simulink model "lab7_1"  (R2018b)
settings: Solver=VariableStepAuto  StartTime=0.0  StopTime=10.0  RelTol=1e-3
libraries: hdlsllib x86
(part 1 of 2)
settings Model: Creator=Patrick  LastModifiedBy=Patrick

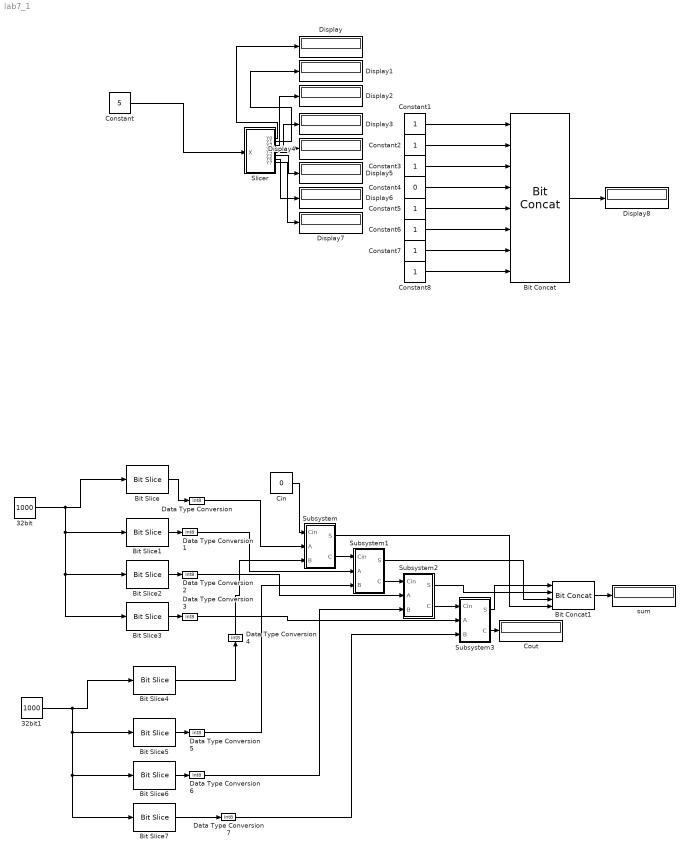
== system lab7_1 ==
  32bit : Constant  Value=1000  OutDataTypeStr=int32  SampleTime=1
  32bit1 : Constant  Value=1000  OutDataTypeStr=int32  SampleTime=1
  Bit Concat : hdlsllib/Logic and Bit Operations/Bit Concat  numInputs=8
      settings: SourceProductName=HDL Coder  SourceProductBaseCode=HD
  Bit Concat1 : hdlsllib/Logic and Bit Operations/Bit Concat  numInputs=4
      settings: SourceProductName=HDL Coder  SourceProductBaseCode=HD
  Bit Slice : hdlsllib/Logic and Bit Operations/Bit Slice  lidx=7  ridx=0
  Bit Slice1 : hdlsllib/Logic and Bit Operations/Bit Slice  lidx=15  ridx=8
  Bit Slice2 : hdlsllib/Logic and Bit Operations/Bit Slice  lidx=23  ridx=16
  Bit Slice3 : hdlsllib/Logic and Bit Operations/Bit Slice  lidx=31  ridx=24
  Bit Slice4 : hdlsllib/Logic and Bit Operations/Bit Slice  lidx=7  ridx=0
  Bit Slice5 : hdlsllib/Logic and Bit Operations/Bit Slice  lidx=15  ridx=8
  Bit Slice6 : hdlsllib/Logic and Bit Operations/Bit Slice  lidx=23  ridx=16
  Bit Slice7 : hdlsllib/Logic and Bit Operations/Bit Slice  lidx=31  ridx=24
  Cin : Constant  Value=0  OutDataTypeStr=boolean  SampleTime=1
  Constant : Constant  Value=5  OutDataTypeStr=int8
  Constant{1..3,5..8} (7 alike) : Constant  OutDataTypeStr=boolean
  Constant4 : Constant  Value=0  OutDataTypeStr=boolean
  Cout : Display
  Data Type Conversion{,1..7} (8 alike) : DataTypeConversion  OutDataTypeStr=int8
  Display{,1..8} (9 alike) : Display
  Slicer : Subsystem
  Subsystem : Subsystem
  Subsystem1 : Subsystem
  Subsystem2 : Subsystem
  Subsystem3 : Subsystem
  sum : Display
  wires:
  Constant/1 -> Slicer/1(X)
  Slicer/8(Y7) -> Display7/1
  Slicer/7(Y6) -> Display6/1
  Slicer/6(Y5) -> Display5/1
  Slicer/5(Y4) -> Display4/1
  Slicer/4(Y3) -> Display3/1
  Slicer/3(Y2) -> Display2/1
  Slicer/2(Y1) -> Display1/1
  Slicer/1(Y0) -> Display/1
  Constant1/1 -> Bit Concat/1
  Constant2/1 -> Bit Concat/2
  Constant3/1 -> Bit Concat/3
  Constant4/1 -> Bit Concat/4
  Constant5/1 -> Bit Concat/5
  Constant6/1 -> Bit Concat/6
  Constant7/1 -> Bit Concat/7
  Constant8/1 -> Bit Concat/8
  Bit Concat/1 -> Display8/1
  32bit/1 -> Bit Slice3/1, Bit Slice2/1, Bit Slice1/1, Bit Slice/1
  Bit Slice/1 -> Data Type Conversion/1
  Bit Slice2/1 -> Data Type Conversion2/1
  Bit Slice3/1 -> Data Type Conversion3/1
  Subsystem2/2(C) -> Subsystem3/1(Cin)
  Subsystem1/2(C) -> Subsystem2/1(Cin)
  Subsystem/2(C) -> Subsystem1/1(Cin)
  Bit Slice4/1 -> Data Type Conversion4/1
  32bit1/1 -> Bit Slice7/1, Bit Slice6/1, Bit Slice5/1, Bit Slice4/1
  Bit Slice7/1 -> Data Type Conversion7/1
  Subsystem3/1(S) -> Bit Concat1/1
  Subsystem2/1(S) -> Bit Concat1/2
  Subsystem1/1(S) -> Bit Concat1/3
  Subsystem/1(S) -> Bit Concat1/4
  Subsystem3/2(C) -> Cout/1
  Bit Concat1/1 -> sum/1
  Cin/1 -> Subsystem/1(Cin)
  Data Type Conversion/1 -> Subsystem/2(A)
  Data Type Conversion7/1 -> Subsystem3/3(B)
  Bit Slice6/1 -> Data Type Conversion6/1
  Data Type Conversion6/1 -> Subsystem2/3(B)
  Bit Slice5/1 -> Data Type Conversion5/1
  Data Type Conversion5/1 -> Subsystem1/3(B)
  Data Type Conversion4/1 -> Subsystem/3(B)
  Data Type Conversion3/1 -> Subsystem3/2(A)
  Data Type Conversion2/1 -> Subsystem2/2(A)
  Bit Slice1/1 -> Data Type Conversion1/1
  Data Type Conversion1/1 -> Subsystem1/2(A)

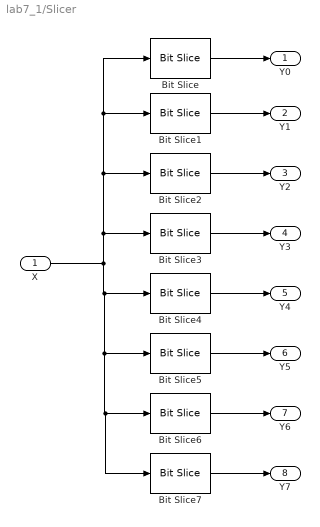
== system lab7_1/Slicer ==
  X : Inport  OutDataTypeStr=int8  SampleTime=1
  Bit Slice : hdlsllib/Logic and Bit Operations/Bit Slice  lidx=7  ridx=7
  Bit Slice1 : hdlsllib/Logic and Bit Operations/Bit Slice  lidx=6  ridx=6
  Bit Slice2 : hdlsllib/Logic and Bit Operations/Bit Slice  lidx=5  ridx=5
  Bit Slice3 : hdlsllib/Logic and Bit Operations/Bit Slice  lidx=4  ridx=4
  Bit Slice4 : hdlsllib/Logic and Bit Operations/Bit Slice  lidx=3  ridx=3
  Bit Slice5 : hdlsllib/Logic and Bit Operations/Bit Slice  lidx=2  ridx=2
  Bit Slice6 : hdlsllib/Logic and Bit Operations/Bit Slice  lidx=1  ridx=1
  Bit Slice7 : hdlsllib/Logic and Bit Operations/Bit Slice  lidx=0  ridx=0
  Y0 : Outport
  Y1 : Outport  Port=2
  Y2 : Outport  Port=3
  Y3 : Outport  Port=4
  Y4 : Outport  Port=5
  Y5 : Outport  Port=6
  Y6 : Outport  Port=7
  Y7 : Outport  Port=8
  wires:
  Bit Slice1/1 -> Y1/1
  Bit Slice7/1 -> Y7/1
  X/1 -> Bit Slice7/1, Bit Slice6/1, Bit Slice5/1, Bit Slice4/1, Bit Slice3/1, Bit Slice2/1, Bit Slice1/1, Bit Slice/1
  Bit Slice/1 -> Y0/1
  Bit Slice4/1 -> Y4/1
  Bit Slice2/1 -> Y2/1
  Bit Slice5/1 -> Y5/1
  Bit Slice3/1 -> Y3/1
  Bit Slice6/1 -> Y6/1

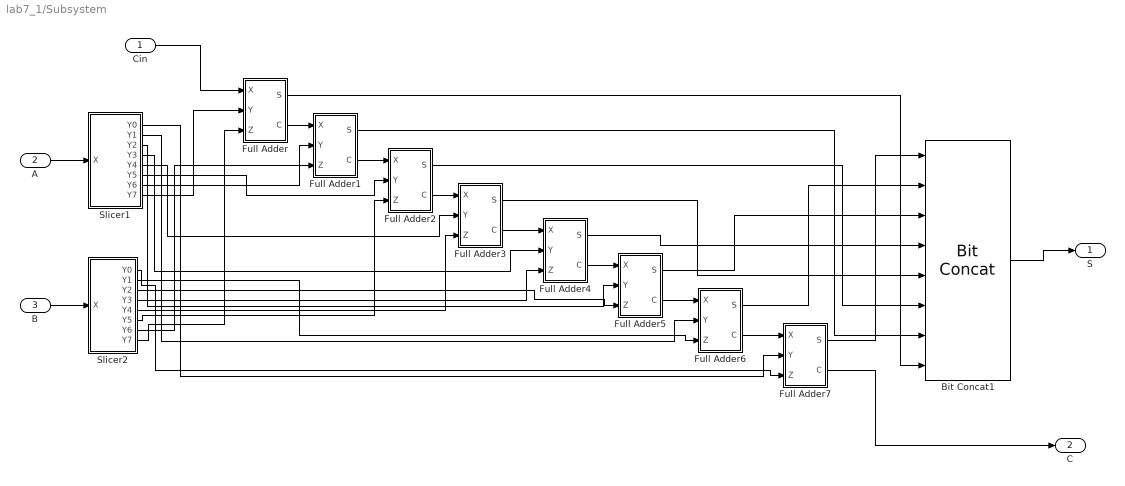
== system lab7_1/Subsystem ==
  Cin : Inport
  A : Inport  Port=2  OutDataTypeStr=int8
  B : Inport  Port=3  OutDataTypeStr=int8
  Bit Concat1 : hdlsllib/Logic and Bit Operations/Bit Concat  numInputs=8
      settings: SourceProductName=HDL Coder  SourceProductBaseCode=HD
  Full Adder : Subsystem
  Full Adder1 : Subsystem
  Full Adder2 : Subsystem
  Full Adder3 : Subsystem
  Full Adder4 : Subsystem
  Full Adder5 : Subsystem
  Full Adder6 : Subsystem
  Full Adder7 : Subsystem
  Slicer1 : Subsystem
  Slicer2 : Subsystem
  S : Outport
  C : Outport  Port=2
  wires:
  Full Adder/1(S) -> Bit Concat1/8
  A/1 -> Slicer1/1(X)
  Slicer1/8(Y7) -> Full Adder/2(Y)
  Cin/1 -> Full Adder/1(X)
  Full Adder4/2(C) -> Full Adder5/1(X)
  Slicer2/1(Y0) -> Full Adder7/3(Z)
  B/1 -> Slicer2/1(X)
  Slicer1/4(Y3) -> Full Adder4/2(Y)
  Slicer2/8(Y7) -> Full Adder/3(Z)
  Full Adder5/1(S) -> Bit Concat1/3
  Full Adder3/2(C) -> Full Adder4/1(X)
  Full Adder5/2(C) -> Full Adder6/1(X)
  Full Adder4/1(S) -> Bit Concat1/4
  Full Adder6/1(S) -> Bit Concat1/2
  Full Adder7/2(C) -> C/1
  Bit Concat1/1 -> S/1
  Slicer2/6(Y5) -> Full Adder2/3(Z)
  Slicer2/4(Y3) -> Full Adder4/3(Z)
  Full Adder7/1(S) -> Bit Concat1/1
  Full Adder/2(C) -> Full Adder1/1(X)
  Full Adder2/2(C) -> Full Adder3/1(X)
  Full Adder6/2(C) -> Full Adder7/1(X)
  Slicer1/5(Y4) -> Full Adder3/2(Y)
  Full Adder3/1(S) -> Bit Concat1/5
  Slicer2/7(Y6) -> Full Adder1/3(Z)
  Slicer2/2(Y1) -> Full Adder6/3(Z)
  Slicer1/1(Y0) -> Full Adder7/2(Y)
  Slicer2/5(Y4) -> Full Adder3/3(Z)
  Full Adder1/2(C) -> Full Adder2/1(X)
  Full Adder2/1(S) -> Bit Concat1/6
  Slicer1/6(Y5) -> Full Adder2/2(Y)
  Full Adder1/1(S) -> Bit Concat1/7
  Slicer1/3(Y2) -> Full Adder5/2(Y)
  Slicer1/7(Y6) -> Full Adder1/2(Y)
  Slicer2/3(Y2) -> Full Adder5/3(Z)
  Slicer1/2(Y1) -> Full Adder6/2(Y)

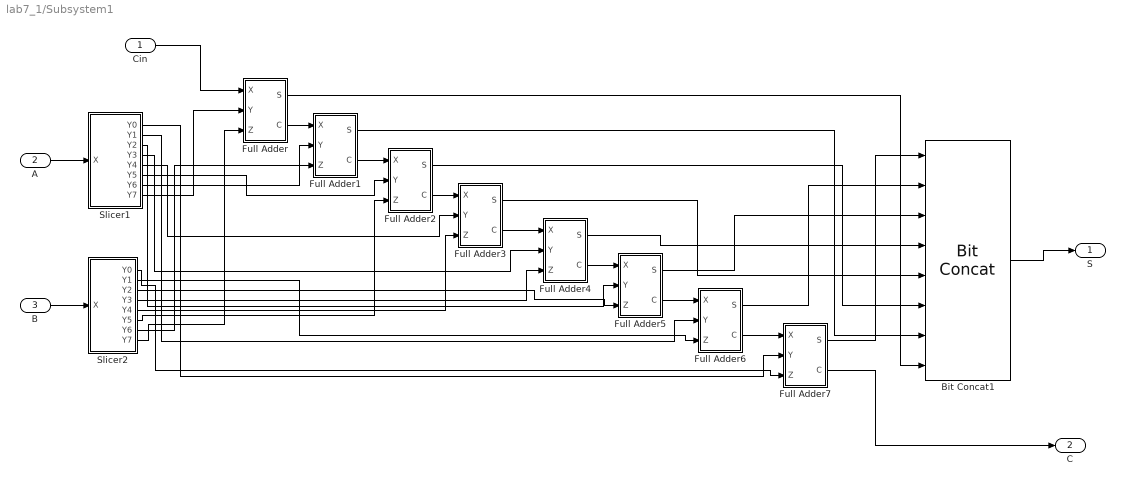
== system lab7_1/Subsystem1 ==
  Cin : Inport
  A : Inport  Port=2
  B : Inport  Port=3
  Bit Concat1 : hdlsllib/Logic and Bit Operations/Bit Concat  numInputs=8
      settings: SourceProductName=HDL Coder  SourceProductBaseCode=HD
  Full Adder : Subsystem
  Full Adder1 : Subsystem
  Full Adder2 : Subsystem
  Full Adder3 : Subsystem
  Full Adder4 : Subsystem
  Full Adder5 : Subsystem
  Full Adder6 : Subsystem
  Full Adder7 : Subsystem
  Slicer1 : Subsystem
  Slicer2 : Subsystem
  S : Outport
  C : Outport  Port=2
  wires:
  Full Adder/1(S) -> Bit Concat1/8
  A/1 -> Slicer1/1(X)
  Slicer1/8(Y7) -> Full Adder/2(Y)
  Cin/1 -> Full Adder/1(X)
  Full Adder4/2(C) -> Full Adder5/1(X)
  Slicer2/1(Y0) -> Full Adder7/3(Z)
  B/1 -> Slicer2/1(X)
  Slicer1/4(Y3) -> Full Adder4/2(Y)
  Slicer2/8(Y7) -> Full Adder/3(Z)
  Full Adder5/1(S) -> Bit Concat1/3
  Full Adder3/2(C) -> Full Adder4/1(X)
  Full Adder5/2(C) -> Full Adder6/1(X)
  Full Adder4/1(S) -> Bit Concat1/4
  Full Adder6/1(S) -> Bit Concat1/2
  Full Adder7/2(C) -> C/1
  Bit Concat1/1 -> S/1
  Slicer2/6(Y5) -> Full Adder2/3(Z)
  Slicer2/4(Y3) -> Full Adder4/3(Z)
  Full Adder7/1(S) -> Bit Concat1/1
  Full Adder/2(C) -> Full Adder1/1(X)
  Full Adder2/2(C) -> Full Adder3/1(X)
  Full Adder6/2(C) -> Full Adder7/1(X)
  Slicer1/5(Y4) -> Full Adder3/2(Y)
  Full Adder3/1(S) -> Bit Concat1/5
  Slicer2/7(Y6) -> Full Adder1/3(Z)
  Slicer2/2(Y1) -> Full Adder6/3(Z)
  Slicer1/1(Y0) -> Full Adder7/2(Y)
  Slicer2/5(Y4) -> Full Adder3/3(Z)
  Full Adder1/2(C) -> Full Adder2/1(X)
  Full Adder2/1(S) -> Bit Concat1/6
  Slicer1/6(Y5) -> Full Adder2/2(Y)
  Full Adder1/1(S) -> Bit Concat1/7
  Slicer1/3(Y2) -> Full Adder5/2(Y)
  Slicer1/7(Y6) -> Full Adder1/2(Y)
  Slicer2/3(Y2) -> Full Adder5/3(Z)
  Slicer1/2(Y1) -> Full Adder6/2(Y)

== system lab7_1/Subsystem2 ==
  Cin : Inport
  A : Inport  Port=2
  B : Inport  Port=3
  Bit Concat1 : hdlsllib/Logic and Bit Operations/Bit Concat  numInputs=8
      settings: SourceProductName=HDL Coder  SourceProductBaseCode=HD
  Full Adder : Subsystem
  Full Adder1 : Subsystem
  Full Adder2 : Subsystem
  Full Adder3 : Subsystem
  Full Adder4 : Subsystem
  Full Adder5 : Subsystem
  Full Adder6 : Subsystem
  Full Adder7 : Subsystem
  Slicer1 : Subsystem
  Slicer2 : Subsystem
  S : Outport
  C : Outport  Port=2
  wires:
  Full Adder/1(S) -> Bit Concat1/8
  A/1 -> Slicer1/1(X)
  Slicer1/8(Y7) -> Full Adder/2(Y)
  Cin/1 -> Full Adder/1(X)
  Full Adder4/2(C) -> Full Adder5/1(X)
  Slicer2/1(Y0) -> Full Adder7/3(Z)
  B/1 -> Slicer2/1(X)
  Slicer1/4(Y3) -> Full Adder4/2(Y)
  Slicer2/8(Y7) -> Full Adder/3(Z)
  Full Adder5/1(S) -> Bit Concat1/3
  Full Adder3/2(C) -> Full Adder4/1(X)
  Full Adder5/2(C) -> Full Adder6/1(X)
  Full Adder4/1(S) -> Bit Concat1/4
  Full Adder6/1(S) -> Bit Concat1/2
  Full Adder7/2(C) -> C/1
  Bit Concat1/1 -> S/1
  Slicer2/6(Y5) -> Full Adder2/3(Z)
  Slicer2/4(Y3) -> Full Adder4/3(Z)
  Full Adder7/1(S) -> Bit Concat1/1
  Full Adder/2(C) -> Full Adder1/1(X)
  Full Adder2/2(C) -> Full Adder3/1(X)
  Full Adder6/2(C) -> Full Adder7/1(X)
  Slicer1/5(Y4) -> Full Adder3/2(Y)
  Full Adder3/1(S) -> Bit Concat1/5
  Slicer2/7(Y6) -> Full Adder1/3(Z)
  Slicer2/2(Y1) -> Full Adder6/3(Z)
  Slicer1/1(Y0) -> Full Adder7/2(Y)
  Slicer2/5(Y4) -> Full Adder3/3(Z)
  Full Adder1/2(C) -> Full Adder2/1(X)
  Full Adder2/1(S) -> Bit Concat1/6
  Slicer1/6(Y5) -> Full Adder2/2(Y)
  Full Adder1/1(S) -> Bit Concat1/7
  Slicer1/3(Y2) -> Full Adder5/2(Y)
  Slicer1/7(Y6) -> Full Adder1/2(Y)
  Slicer2/3(Y2) -> Full Adder5/3(Z)
  Slicer1/2(Y1) -> Full Adder6/2(Y)

== system lab7_1/Subsystem3 ==
  Cin : Inport
  A : Inport  Port=2
  B : Inport  Port=3
  Bit Concat1 : hdlsllib/Logic and Bit Operations/Bit Concat  numInputs=8
      settings: SourceProductName=HDL Coder  SourceProductBaseCode=HD
  Full Adder : Subsystem
  Full Adder1 : Subsystem
  Full Adder2 : Subsystem
  Full Adder3 : Subsystem
  Full Adder4 : Subsystem
  Full Adder5 : Subsystem
  Full Adder6 : Subsystem
  Full Adder7 : Subsystem
  Slicer1 : Subsystem
  Slicer2 : Subsystem
  S : Outport
  C : Outport  Port=2
  wires:
  Full Adder/1(S) -> Bit Concat1/8
  A/1 -> Slicer1/1(X)
  Slicer1/8(Y7) -> Full Adder/2(Y)
  Cin/1 -> Full Adder/1(X)
  Full Adder4/2(C) -> Full Adder5/1(X)
  Slicer2/1(Y0) -> Full Adder7/3(Z)
  B/1 -> Slicer2/1(X)
  Slicer1/4(Y3) -> Full Adder4/2(Y)
  Slicer2/8(Y7) -> Full Adder/3(Z)
  Full Adder5/1(S) -> Bit Concat1/3
  Full Adder3/2(C) -> Full Adder4/1(X)
  Full Adder5/2(C) -> Full Adder6/1(X)
  Full Adder4/1(S) -> Bit Concat1/4
  Full Adder6/1(S) -> Bit Concat1/2
  Full Adder7/2(C) -> C/1
  Bit Concat1/1 -> S/1
  Slicer2/6(Y5) -> Full Adder2/3(Z)
  Slicer2/4(Y3) -> Full Adder4/3(Z)
  Full Adder7/1(S) -> Bit Concat1/1
  Full Adder/2(C) -> Full Adder1/1(X)
  Full Adder2/2(C) -> Full Adder3/1(X)
  Full Adder6/2(C) -> Full Adder7/1(X)
  Slicer1/5(Y4) -> Full Adder3/2(Y)
  Full Adder3/1(S) -> Bit Concat1/5
  Slicer2/7(Y6) -> Full Adder1/3(Z)
  Slicer2/2(Y1) -> Full Adder6/3(Z)
  Slicer1/1(Y0) -> Full Adder7/2(Y)
  Slicer2/5(Y4) -> Full Adder3/3(Z)
  Full Adder1/2(C) -> Full Adder2/1(X)
  Full Adder2/1(S) -> Bit Concat1/6
  Slicer1/6(Y5) -> Full Adder2/2(Y)
  Full Adder1/1(S) -> Bit Concat1/7
  Slicer1/3(Y2) -> Full Adder5/2(Y)
  Slicer1/7(Y6) -> Full Adder1/2(Y)
  Slicer2/3(Y2) -> Full Adder5/3(Z)
  Slicer1/2(Y1) -> Full Adder6/2(Y)

== system lab7_1/Subsystem/Full Adder ==
  X : Inport
  Y : Inport  Port=2
  Z : Inport  Port=3
  Half Adder : Subsystem
  Half Adder 1 : Subsystem
  Logical Operator : Logic  Operator=OR  IconShape=distinctive  AllPortsSameDT=off  OutDataTypeStr=boolean
  S : Outport
  C : Outport  Port=2
  wires:
  Half Adder/1(S) -> Half Adder 1/1(X)
  Y/1 -> Half Adder/2(Y)
  Half Adder 1/2(C) -> Logical Operator/1
  Z/1 -> Half Adder 1/2(Y)
  Half Adder/2(C) -> Logical Operator/2
  X/1 -> Half Adder/1(X)
  Half Adder 1/1(S) -> S/1
  Logical Operator/1 -> C/1

== system lab7_1/Subsystem/Full Adder1 ==
  X : Inport
  Y : Inport  Port=2
  Z : Inport  Port=3
  Half Adder : Subsystem
  Half Adder 1 : Subsystem
  Logical Operator : Logic  Operator=OR  IconShape=distinctive  AllPortsSameDT=off  OutDataTypeStr=boolean
  S : Outport
  C : Outport  Port=2
  wires:
  Half Adder/1(S) -> Half Adder 1/1(X)
  Y/1 -> Half Adder/2(Y)
  Half Adder 1/2(C) -> Logical Operator/1
  Z/1 -> Half Adder 1/2(Y)
  Half Adder/2(C) -> Logical Operator/2
  X/1 -> Half Adder/1(X)
  Half Adder 1/1(S) -> S/1
  Logical Operator/1 -> C/1

== system lab7_1/Subsystem/Full Adder2 ==
  X : Inport
  Y : Inport  Port=2
  Z : Inport  Port=3
  Half Adder : Subsystem
  Half Adder 1 : Subsystem
  Logical Operator : Logic  Operator=OR  IconShape=distinctive  AllPortsSameDT=off  OutDataTypeStr=boolean
  S : Outport
  C : Outport  Port=2
  wires:
  Half Adder/1(S) -> Half Adder 1/1(X)
  Y/1 -> Half Adder/2(Y)
  Half Adder 1/2(C) -> Logical Operator/1
  Z/1 -> Half Adder 1/2(Y)
  Half Adder/2(C) -> Logical Operator/2
  X/1 -> Half Adder/1(X)
  Half Adder 1/1(S) -> S/1
  Logical Operator/1 -> C/1

== system lab7_1/Subsystem/Full Adder3 ==
  X : Inport
  Y : Inport  Port=2
  Z : Inport  Port=3
  Half Adder : Subsystem
  Half Adder 1 : Subsystem
  Logical Operator : Logic  Operator=OR  IconShape=distinctive  AllPortsSameDT=off  OutDataTypeStr=boolean
  S : Outport
  C : Outport  Port=2
  wires:
  Half Adder/1(S) -> Half Adder 1/1(X)
  Y/1 -> Half Adder/2(Y)
  Half Adder 1/2(C) -> Logical Operator/1
  Z/1 -> Half Adder 1/2(Y)
  Half Adder/2(C) -> Logical Operator/2
  X/1 -> Half Adder/1(X)
  Half Adder 1/1(S) -> S/1
  Logical Operator/1 -> C/1

== system lab7_1/Subsystem/Full Adder4 ==
  X : Inport
  Y : Inport  Port=2
  Z : Inport  Port=3
  Half Adder : Subsystem
  Half Adder 1 : Subsystem
  Logical Operator : Logic  Operator=OR  IconShape=distinctive  AllPortsSameDT=off  OutDataTypeStr=boolean
  S : Outport
  C : Outport  Port=2
  wires:
  Half Adder/1(S) -> Half Adder 1/1(X)
  Y/1 -> Half Adder/2(Y)
  Half Adder 1/2(C) -> Logical Operator/1
  Z/1 -> Half Adder 1/2(Y)
  Half Adder/2(C) -> Logical Operator/2
  X/1 -> Half Adder/1(X)
  Half Adder 1/1(S) -> S/1
  Logical Operator/1 -> C/1

== system lab7_1/Subsystem/Full Adder5 ==
  X : Inport
  Y : Inport  Port=2
  Z : Inport  Port=3
  Half Adder : Subsystem
  Half Adder 1 : Subsystem
  Logical Operator : Logic  Operator=OR  IconShape=distinctive  AllPortsSameDT=off  OutDataTypeStr=boolean
  S : Outport
  C : Outport  Port=2
  wires:
  Half Adder/1(S) -> Half Adder 1/1(X)
  Y/1 -> Half Adder/2(Y)
  Half Adder 1/2(C) -> Logical Operator/1
  Z/1 -> Half Adder 1/2(Y)
  Half Adder/2(C) -> Logical Operator/2
  X/1 -> Half Adder/1(X)
  Half Adder 1/1(S) -> S/1
  Logical Operator/1 -> C/1

== system lab7_1/Subsystem/Full Adder6 ==
  X : Inport
  Y : Inport  Port=2
  Z : Inport  Port=3
  Half Adder : Subsystem
  Half Adder 1 : Subsystem
  Logical Operator : Logic  Operator=OR  IconShape=distinctive  AllPortsSameDT=off  OutDataTypeStr=boolean
  S : Outport
  C : Outport  Port=2
  wires:
  Half Adder/1(S) -> Half Adder 1/1(X)
  Y/1 -> Half Adder/2(Y)
  Half Adder 1/2(C) -> Logical Operator/1
  Z/1 -> Half Adder 1/2(Y)
  Half Adder/2(C) -> Logical Operator/2
  X/1 -> Half Adder/1(X)
  Half Adder 1/1(S) -> S/1
  Logical Operator/1 -> C/1

== system lab7_1/Subsystem/Full Adder7 ==
  X : Inport
  Y : Inport  Port=2
  Z : Inport  Port=3
  Half Adder : Subsystem
  Half Adder 1 : Subsystem
  Logical Operator : Logic  Operator=OR  IconShape=distinctive  AllPortsSameDT=off  OutDataTypeStr=boolean
  S : Outport
  C : Outport  Port=2
  wires:
  Half Adder/1(S) -> Half Adder 1/1(X)
  Y/1 -> Half Adder/2(Y)
  Half Adder 1/2(C) -> Logical Operator/1
  Z/1 -> Half Adder 1/2(Y)
  Half Adder/2(C) -> Logical Operator/2
  X/1 -> Half Adder/1(X)
  Half Adder 1/1(S) -> S/1
  Logical Operator/1 -> C/1

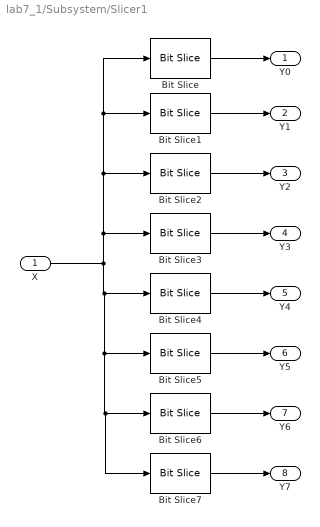
== system lab7_1/Subsystem/Slicer1 ==
  X : Inport  OutDataTypeStr=int8  SampleTime=1
  Bit Slice : hdlsllib/Logic and Bit Operations/Bit Slice  lidx=7  ridx=7
  Bit Slice1 : hdlsllib/Logic and Bit Operations/Bit Slice  lidx=6  ridx=6
  Bit Slice2 : hdlsllib/Logic and Bit Operations/Bit Slice  lidx=5  ridx=5
  Bit Slice3 : hdlsllib/Logic and Bit Operations/Bit Slice  lidx=4  ridx=4
  Bit Slice4 : hdlsllib/Logic and Bit Operations/Bit Slice  lidx=3  ridx=3
  Bit Slice5 : hdlsllib/Logic and Bit Operations/Bit Slice  lidx=2  ridx=2
  Bit Slice6 : hdlsllib/Logic and Bit Operations/Bit Slice  lidx=1  ridx=1
  Bit Slice7 : hdlsllib/Logic and Bit Operations/Bit Slice  lidx=0  ridx=0
  Y0 : Outport
  Y1 : Outport  Port=2
  Y2 : Outport  Port=3
  Y3 : Outport  Port=4
  Y4 : Outport  Port=5
  Y5 : Outport  Port=6
  Y6 : Outport  Port=7
  Y7 : Outport  Port=8
  wires:
  Bit Slice1/1 -> Y1/1
  Bit Slice7/1 -> Y7/1
  X/1 -> Bit Slice7/1, Bit Slice6/1, Bit Slice5/1, Bit Slice4/1, Bit Slice3/1, Bit Slice2/1, Bit Slice1/1, Bit Slice/1
  Bit Slice/1 -> Y0/1
  Bit Slice4/1 -> Y4/1
  Bit Slice2/1 -> Y2/1
  Bit Slice5/1 -> Y5/1
  Bit Slice3/1 -> Y3/1
  Bit Slice6/1 -> Y6/1

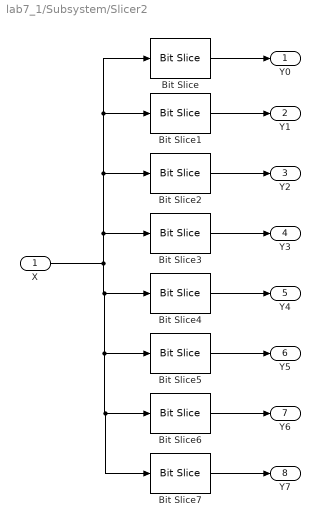
== system lab7_1/Subsystem/Slicer2 ==
  X : Inport  OutDataTypeStr=int8  SampleTime=1
  Bit Slice : hdlsllib/Logic and Bit Operations/Bit Slice  lidx=7  ridx=7
  Bit Slice1 : hdlsllib/Logic and Bit Operations/Bit Slice  lidx=6  ridx=6
  Bit Slice2 : hdlsllib/Logic and Bit Operations/Bit Slice  lidx=5  ridx=5
  Bit Slice3 : hdlsllib/Logic and Bit Operations/Bit Slice  lidx=4  ridx=4
  Bit Slice4 : hdlsllib/Logic and Bit Operations/Bit Slice  lidx=3  ridx=3
  Bit Slice5 : hdlsllib/Logic and Bit Operations/Bit Slice  lidx=2  ridx=2
  Bit Slice6 : hdlsllib/Logic and Bit Operations/Bit Slice  lidx=1  ridx=1
  Bit Slice7 : hdlsllib/Logic and Bit Operations/Bit Slice  lidx=0  ridx=0
  Y0 : Outport
  Y1 : Outport  Port=2
  Y2 : Outport  Port=3
  Y3 : Outport  Port=4
  Y4 : Outport  Port=5
  Y5 : Outport  Port=6
  Y6 : Outport  Port=7
  Y7 : Outport  Port=8
  wires:
  Bit Slice1/1 -> Y1/1
  Bit Slice7/1 -> Y7/1
  X/1 -> Bit Slice7/1, Bit Slice6/1, Bit Slice5/1, Bit Slice4/1, Bit Slice3/1, Bit Slice2/1, Bit Slice1/1, Bit Slice/1
  Bit Slice/1 -> Y0/1
  Bit Slice4/1 -> Y4/1
  Bit Slice2/1 -> Y2/1
  Bit Slice5/1 -> Y5/1
  Bit Slice3/1 -> Y3/1
  Bit Slice6/1 -> Y6/1

== system lab7_1/Subsystem1/Full Adder ==
  X : Inport
  Y : Inport  Port=2
  Z : Inport  Port=3
  Half Adder : Subsystem
  Half Adder 1 : Subsystem
  Logical Operator : Logic  Operator=OR  IconShape=distinctive  AllPortsSameDT=off  OutDataTypeStr=boolean
  S : Outport
  C : Outport  Port=2
  wires:
  Half Adder/1(S) -> Half Adder 1/1(X)
  Y/1 -> Half Adder/2(Y)
  Half Adder 1/2(C) -> Logical Operator/1
  Z/1 -> Half Adder 1/2(Y)
  Half Adder/2(C) -> Logical Operator/2
  X/1 -> Half Adder/1(X)
  Half Adder 1/1(S) -> S/1
  Logical Operator/1 -> C/1

== system lab7_1/Subsystem1/Full Adder1 ==
  X : Inport
  Y : Inport  Port=2
  Z : Inport  Port=3
  Half Adder : Subsystem
  Half Adder 1 : Subsystem
  Logical Operator : Logic  Operator=OR  IconShape=distinctive  AllPortsSameDT=off  OutDataTypeStr=boolean
  S : Outport
  C : Outport  Port=2
  wires:
  Half Adder/1(S) -> Half Adder 1/1(X)
  Y/1 -> Half Adder/2(Y)
  Half Adder 1/2(C) -> Logical Operator/1
  Z/1 -> Half Adder 1/2(Y)
  Half Adder/2(C) -> Logical Operator/2
  X/1 -> Half Adder/1(X)
  Half Adder 1/1(S) -> S/1
  Logical Operator/1 -> C/1

== system lab7_1/Subsystem1/Full Adder2 ==
  X : Inport
  Y : Inport  Port=2
  Z : Inport  Port=3
  Half Adder : Subsystem
  Half Adder 1 : Subsystem
  Logical Operator : Logic  Operator=OR  IconShape=distinctive  AllPortsSameDT=off  OutDataTypeStr=boolean
  S : Outport
  C : Outport  Port=2
  wires:
  Half Adder/1(S) -> Half Adder 1/1(X)
  Y/1 -> Half Adder/2(Y)
  Half Adder 1/2(C) -> Logical Operator/1
  Z/1 -> Half Adder 1/2(Y)
  Half Adder/2(C) -> Logical Operator/2
  X/1 -> Half Adder/1(X)
  Half Adder 1/1(S) -> S/1
  Logical Operator/1 -> C/1

== system lab7_1/Subsystem1/Full Adder3 ==
  X : Inport
  Y : Inport  Port=2
  Z : Inport  Port=3
  Half Adder : Subsystem
  Half Adder 1 : Subsystem
  Logical Operator : Logic  Operator=OR  IconShape=distinctive  AllPortsSameDT=off  OutDataTypeStr=boolean
  S : Outport
  C : Outport  Port=2
  wires:
  Half Adder/1(S) -> Half Adder 1/1(X)
  Y/1 -> Half Adder/2(Y)
  Half Adder 1/2(C) -> Logical Operator/1
  Z/1 -> Half Adder 1/2(Y)
  Half Adder/2(C) -> Logical Operator/2
  X/1 -> Half Adder/1(X)
  Half Adder 1/1(S) -> S/1
  Logical Operator/1 -> C/1

== system lab7_1/Subsystem1/Full Adder4 ==
  X : Inport
  Y : Inport  Port=2
  Z : Inport  Port=3
  Half Adder : Subsystem
  Half Adder 1 : Subsystem
  Logical Operator : Logic  Operator=OR  IconShape=distinctive  AllPortsSameDT=off  OutDataTypeStr=boolean
  S : Outport
  C : Outport  Port=2
  wires:
  Half Adder/1(S) -> Half Adder 1/1(X)
  Y/1 -> Half Adder/2(Y)
  Half Adder 1/2(C) -> Logical Operator/1
  Z/1 -> Half Adder 1/2(Y)
  Half Adder/2(C) -> Logical Operator/2
  X/1 -> Half Adder/1(X)
  Half Adder 1/1(S) -> S/1
  Logical Operator/1 -> C/1

== system lab7_1/Subsystem1/Full Adder5 ==
  X : Inport
  Y : Inport  Port=2
  Z : Inport  Port=3
  Half Adder : Subsystem
  Half Adder 1 : Subsystem
  Logical Operator : Logic  Operator=OR  IconShape=distinctive  AllPortsSameDT=off  OutDataTypeStr=boolean
  S : Outport
  C : Outport  Port=2
  wires:
  Half Adder/1(S) -> Half Adder 1/1(X)
  Y/1 -> Half Adder/2(Y)
  Half Adder 1/2(C) -> Logical Operator/1
  Z/1 -> Half Adder 1/2(Y)
  Half Adder/2(C) -> Logical Operator/2
  X/1 -> Half Adder/1(X)
  Half Adder 1/1(S) -> S/1
  Logical Operator/1 -> C/1

== system lab7_1/Subsystem1/Full Adder6 ==
  X : Inport
  Y : Inport  Port=2
  Z : Inport  Port=3
  Half Adder : Subsystem
  Half Adder 1 : Subsystem
  Logical Operator : Logic  Operator=OR  IconShape=distinctive  AllPortsSameDT=off  OutDataTypeStr=boolean
  S : Outport
  C : Outport  Port=2
  wires:
  Half Adder/1(S) -> Half Adder 1/1(X)
  Y/1 -> Half Adder/2(Y)
  Half Adder 1/2(C) -> Logical Operator/1
  Z/1 -> Half Adder 1/2(Y)
  Half Adder/2(C) -> Logical Operator/2
  X/1 -> Half Adder/1(X)
  Half Adder 1/1(S) -> S/1
  Logical Operator/1 -> C/1

== system lab7_1/Subsystem1/Full Adder7 ==
  X : Inport
  Y : Inport  Port=2
  Z : Inport  Port=3
  Half Adder : Subsystem
  Half Adder 1 : Subsystem
  Logical Operator : Logic  Operator=OR  IconShape=distinctive  AllPortsSameDT=off  OutDataTypeStr=boolean
  S : Outport
  C : Outport  Port=2
  wires:
  Half Adder/1(S) -> Half Adder 1/1(X)
  Y/1 -> Half Adder/2(Y)
  Half Adder 1/2(C) -> Logical Operator/1
  Z/1 -> Half Adder 1/2(Y)
  Half Adder/2(C) -> Logical Operator/2
  X/1 -> Half Adder/1(X)
  Half Adder 1/1(S) -> S/1
  Logical Operator/1 -> C/1

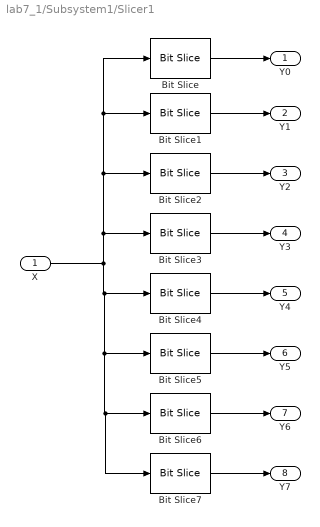
== system lab7_1/Subsystem1/Slicer1 ==
  X : Inport  OutDataTypeStr=int8  SampleTime=1
  Bit Slice : hdlsllib/Logic and Bit Operations/Bit Slice  lidx=7  ridx=7
  Bit Slice1 : hdlsllib/Logic and Bit Operations/Bit Slice  lidx=6  ridx=6
  Bit Slice2 : hdlsllib/Logic and Bit Operations/Bit Slice  lidx=5  ridx=5
  Bit Slice3 : hdlsllib/Logic and Bit Operations/Bit Slice  lidx=4  ridx=4
  Bit Slice4 : hdlsllib/Logic and Bit Operations/Bit Slice  lidx=3  ridx=3
  Bit Slice5 : hdlsllib/Logic and Bit Operations/Bit Slice  lidx=2  ridx=2
  Bit Slice6 : hdlsllib/Logic and Bit Operations/Bit Slice  lidx=1  ridx=1
  Bit Slice7 : hdlsllib/Logic and Bit Operations/Bit Slice  lidx=0  ridx=0
  Y0 : Outport
  Y1 : Outport  Port=2
  Y2 : Outport  Port=3
  Y3 : Outport  Port=4
  Y4 : Outport  Port=5
  Y5 : Outport  Port=6
  Y6 : Outport  Port=7
  Y7 : Outport  Port=8
  wires:
  Bit Slice1/1 -> Y1/1
  Bit Slice7/1 -> Y7/1
  X/1 -> Bit Slice7/1, Bit Slice6/1, Bit Slice5/1, Bit Slice4/1, Bit Slice3/1, Bit Slice2/1, Bit Slice1/1, Bit Slice/1
  Bit Slice/1 -> Y0/1
  Bit Slice4/1 -> Y4/1
  Bit Slice2/1 -> Y2/1
  Bit Slice5/1 -> Y5/1
  Bit Slice3/1 -> Y3/1
  Bit Slice6/1 -> Y6/1

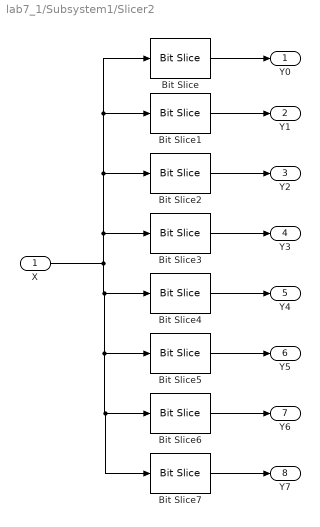
== system lab7_1/Subsystem1/Slicer2 ==
  X : Inport  OutDataTypeStr=int8  SampleTime=1
  Bit Slice : hdlsllib/Logic and Bit Operations/Bit Slice  lidx=7  ridx=7
  Bit Slice1 : hdlsllib/Logic and Bit Operations/Bit Slice  lidx=6  ridx=6
  Bit Slice2 : hdlsllib/Logic and Bit Operations/Bit Slice  lidx=5  ridx=5
  Bit Slice3 : hdlsllib/Logic and Bit Operations/Bit Slice  lidx=4  ridx=4
  Bit Slice4 : hdlsllib/Logic and Bit Operations/Bit Slice  lidx=3  ridx=3
  Bit Slice5 : hdlsllib/Logic and Bit Operations/Bit Slice  lidx=2  ridx=2
  Bit Slice6 : hdlsllib/Logic and Bit Operations/Bit Slice  lidx=1  ridx=1
  Bit Slice7 : hdlsllib/Logic and Bit Operations/Bit Slice  lidx=0  ridx=0
  Y0 : Outport
  Y1 : Outport  Port=2
  Y2 : Outport  Port=3
  Y3 : Outport  Port=4
  Y4 : Outport  Port=5
  Y5 : Outport  Port=6
  Y6 : Outport  Port=7
  Y7 : Outport  Port=8
  wires:
  Bit Slice1/1 -> Y1/1
  Bit Slice7/1 -> Y7/1
  X/1 -> Bit Slice7/1, Bit Slice6/1, Bit Slice5/1, Bit Slice4/1, Bit Slice3/1, Bit Slice2/1, Bit Slice1/1, Bit Slice/1
  Bit Slice/1 -> Y0/1
  Bit Slice4/1 -> Y4/1
  Bit Slice2/1 -> Y2/1
  Bit Slice5/1 -> Y5/1
  Bit Slice3/1 -> Y3/1
  Bit Slice6/1 -> Y6/1

== system lab7_1/Subsystem2/Full Adder ==
  X : Inport
  Y : Inport  Port=2
  Z : Inport  Port=3
  Half Adder : Subsystem
  Half Adder 1 : Subsystem
  Logical Operator : Logic  Operator=OR  IconShape=distinctive  AllPortsSameDT=off  OutDataTypeStr=boolean
  S : Outport
  C : Outport  Port=2
  wires:
  Half Adder/1(S) -> Half Adder 1/1(X)
  Y/1 -> Half Adder/2(Y)
  Half Adder 1/2(C) -> Logical Operator/1
  Z/1 -> Half Adder 1/2(Y)
  Half Adder/2(C) -> Logical Operator/2
  X/1 -> Half Adder/1(X)
  Half Adder 1/1(S) -> S/1
  Logical Operator/1 -> C/1

== system lab7_1/Subsystem2/Full Adder1 ==
  X : Inport
  Y : Inport  Port=2
  Z : Inport  Port=3
  Half Adder : Subsystem
  Half Adder 1 : Subsystem
  Logical Operator : Logic  Operator=OR  IconShape=distinctive  AllPortsSameDT=off  OutDataTypeStr=boolean
  S : Outport
  C : Outport  Port=2
  wires:
  Half Adder/1(S) -> Half Adder 1/1(X)
  Y/1 -> Half Adder/2(Y)
  Half Adder 1/2(C) -> Logical Operator/1
  Z/1 -> Half Adder 1/2(Y)
  Half Adder/2(C) -> Logical Operator/2
  X/1 -> Half Adder/1(X)
  Half Adder 1/1(S) -> S/1
  Logical Operator/1 -> C/1

== system lab7_1/Subsystem2/Full Adder2 ==
  X : Inport
  Y : Inport  Port=2
  Z : Inport  Port=3
  Half Adder : Subsystem
  Half Adder 1 : Subsystem
  Logical Operator : Logic  Operator=OR  IconShape=distinctive  AllPortsSameDT=off  OutDataTypeStr=boolean
  S : Outport
  C : Outport  Port=2
  wires:
  Half Adder/1(S) -> Half Adder 1/1(X)
  Y/1 -> Half Adder/2(Y)
  Half Adder 1/2(C) -> Logical Operator/1
  Z/1 -> Half Adder 1/2(Y)
  Half Adder/2(C) -> Logical Operator/2
  X/1 -> Half Adder/1(X)
  Half Adder 1/1(S) -> S/1
  Logical Operator/1 -> C/1

== system lab7_1/Subsystem2/Full Adder3 ==
  X : Inport
  Y : Inport  Port=2
  Z : Inport  Port=3
  Half Adder : Subsystem
  Half Adder 1 : Subsystem
  Logical Operator : Logic  Operator=OR  IconShape=distinctive  AllPortsSameDT=off  OutDataTypeStr=boolean
  S : Outport
  C : Outport  Port=2
  wires:
  Half Adder/1(S) -> Half Adder 1/1(X)
  Y/1 -> Half Adder/2(Y)
  Half Adder 1/2(C) -> Logical Operator/1
  Z/1 -> Half Adder 1/2(Y)
  Half Adder/2(C) -> Logical Operator/2
  X/1 -> Half Adder/1(X)
  Half Adder 1/1(S) -> S/1
  Logical Operator/1 -> C/1

== system lab7_1/Subsystem2/Full Adder4 ==
  X : Inport
  Y : Inport  Port=2
  Z : Inport  Port=3
  Half Adder : Subsystem
  Half Adder 1 : Subsystem
  Logical Operator : Logic  Operator=OR  IconShape=distinctive  AllPortsSameDT=off  OutDataTypeStr=boolean
  S : Outport
  C : Outport  Port=2
  wires:
  Half Adder/1(S) -> Half Adder 1/1(X)
  Y/1 -> Half Adder/2(Y)
  Half Adder 1/2(C) -> Logical Operator/1
  Z/1 -> Half Adder 1/2(Y)
  Half Adder/2(C) -> Logical Operator/2
  X/1 -> Half Adder/1(X)
  Half Adder 1/1(S) -> S/1
  Logical Operator/1 -> C/1

== system lab7_1/Subsystem2/Full Adder5 ==
  X : Inport
  Y : Inport  Port=2
  Z : Inport  Port=3
  Half Adder : Subsystem
  Half Adder 1 : Subsystem
  Logical Operator : Logic  Operator=OR  IconShape=distinctive  AllPortsSameDT=off  OutDataTypeStr=boolean
  S : Outport
  C : Outport  Port=2
  wires:
  Half Adder/1(S) -> Half Adder 1/1(X)
  Y/1 -> Half Adder/2(Y)
  Half Adder 1/2(C) -> Logical Operator/1
  Z/1 -> Half Adder 1/2(Y)
  Half Adder/2(C) -> Logical Operator/2
  X/1 -> Half Adder/1(X)
  Half Adder 1/1(S) -> S/1
  Logical Operator/1 -> C/1

== system lab7_1/Subsystem2/Full Adder6 ==
  X : Inport
  Y : Inport  Port=2
  Z : Inport  Port=3
  Half Adder : Subsystem
  Half Adder 1 : Subsystem
  Logical Operator : Logic  Operator=OR  IconShape=distinctive  AllPortsSameDT=off  OutDataTypeStr=boolean
  S : Outport
  C : Outport  Port=2
  wires:
  Half Adder/1(S) -> Half Adder 1/1(X)
  Y/1 -> Half Adder/2(Y)
  Half Adder 1/2(C) -> Logical Operator/1
  Z/1 -> Half Adder 1/2(Y)
  Half Adder/2(C) -> Logical Operator/2
  X/1 -> Half Adder/1(X)
  Half Adder 1/1(S) -> S/1
  Logical Operator/1 -> C/1

== system lab7_1/Subsystem2/Full Adder7 ==
  X : Inport
  Y : Inport  Port=2
  Z : Inport  Port=3
  Half Adder : Subsystem
  Half Adder 1 : Subsystem
  Logical Operator : Logic  Operator=OR  IconShape=distinctive  AllPortsSameDT=off  OutDataTypeStr=boolean
  S : Outport
  C : Outport  Port=2
  wires:
  Half Adder/1(S) -> Half Adder 1/1(X)
  Y/1 -> Half Adder/2(Y)
  Half Adder 1/2(C) -> Logical Operator/1
  Z/1 -> Half Adder 1/2(Y)
  Half Adder/2(C) -> Logical Operator/2
  X/1 -> Half Adder/1(X)
  Half Adder 1/1(S) -> S/1
  Logical Operator/1 -> C/1

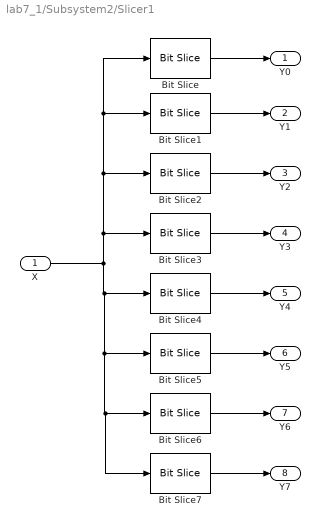
== system lab7_1/Subsystem2/Slicer1 ==
  X : Inport  OutDataTypeStr=int8  SampleTime=1
  Bit Slice : hdlsllib/Logic and Bit Operations/Bit Slice  lidx=7  ridx=7
  Bit Slice1 : hdlsllib/Logic and Bit Operations/Bit Slice  lidx=6  ridx=6
  Bit Slice2 : hdlsllib/Logic and Bit Operations/Bit Slice  lidx=5  ridx=5
  Bit Slice3 : hdlsllib/Logic and Bit Operations/Bit Slice  lidx=4  ridx=4
  Bit Slice4 : hdlsllib/Logic and Bit Operations/Bit Slice  lidx=3  ridx=3
  Bit Slice5 : hdlsllib/Logic and Bit Operations/Bit Slice  lidx=2  ridx=2
  Bit Slice6 : hdlsllib/Logic and Bit Operations/Bit Slice  lidx=1  ridx=1
  Bit Slice7 : hdlsllib/Logic and Bit Operations/Bit Slice  lidx=0  ridx=0
  Y0 : Outport
  Y1 : Outport  Port=2
  Y2 : Outport  Port=3
  Y3 : Outport  Port=4
  Y4 : Outport  Port=5
  Y5 : Outport  Port=6
  Y6 : Outport  Port=7
  Y7 : Outport  Port=8
  wires:
  Bit Slice1/1 -> Y1/1
  Bit Slice7/1 -> Y7/1
  X/1 -> Bit Slice7/1, Bit Slice6/1, Bit Slice5/1, Bit Slice4/1, Bit Slice3/1, Bit Slice2/1, Bit Slice1/1, Bit Slice/1
  Bit Slice/1 -> Y0/1
  Bit Slice4/1 -> Y4/1
  Bit Slice2/1 -> Y2/1
  Bit Slice5/1 -> Y5/1
  Bit Slice3/1 -> Y3/1
  Bit Slice6/1 -> Y6/1

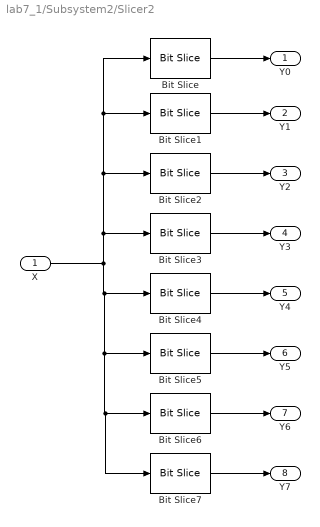
== system lab7_1/Subsystem2/Slicer2 ==
  X : Inport  OutDataTypeStr=int8  SampleTime=1
  Bit Slice : hdlsllib/Logic and Bit Operations/Bit Slice  lidx=7  ridx=7
  Bit Slice1 : hdlsllib/Logic and Bit Operations/Bit Slice  lidx=6  ridx=6
  Bit Slice2 : hdlsllib/Logic and Bit Operations/Bit Slice  lidx=5  ridx=5
  Bit Slice3 : hdlsllib/Logic and Bit Operations/Bit Slice  lidx=4  ridx=4
  Bit Slice4 : hdlsllib/Logic and Bit Operations/Bit Slice  lidx=3  ridx=3
  Bit Slice5 : hdlsllib/Logic and Bit Operations/Bit Slice  lidx=2  ridx=2
  Bit Slice6 : hdlsllib/Logic and Bit Operations/Bit Slice  lidx=1  ridx=1
  Bit Slice7 : hdlsllib/Logic and Bit Operations/Bit Slice  lidx=0  ridx=0
  Y0 : Outport
  Y1 : Outport  Port=2
  Y2 : Outport  Port=3
  Y3 : Outport  Port=4
  Y4 : Outport  Port=5
  Y5 : Outport  Port=6
  Y6 : Outport  Port=7
  Y7 : Outport  Port=8
  wires:
  Bit Slice1/1 -> Y1/1
  Bit Slice7/1 -> Y7/1
  X/1 -> Bit Slice7/1, Bit Slice6/1, Bit Slice5/1, Bit Slice4/1, Bit Slice3/1, Bit Slice2/1, Bit Slice1/1, Bit Slice/1
  Bit Slice/1 -> Y0/1
  Bit Slice4/1 -> Y4/1
  Bit Slice2/1 -> Y2/1
  Bit Slice5/1 -> Y5/1
  Bit Slice3/1 -> Y3/1
  Bit Slice6/1 -> Y6/1

== system lab7_1/Subsystem3/Full Adder ==
  X : Inport
  Y : Inport  Port=2
  Z : Inport  Port=3
  Half Adder : Subsystem
  Half Adder 1 : Subsystem
  Logical Operator : Logic  Operator=OR  IconShape=distinctive  AllPortsSameDT=off  OutDataTypeStr=boolean
  S : Outport
  C : Outport  Port=2
  wires:
  Half Adder/1(S) -> Half Adder 1/1(X)
  Y/1 -> Half Adder/2(Y)
  Half Adder 1/2(C) -> Logical Operator/1
  Z/1 -> Half Adder 1/2(Y)
  Half Adder/2(C) -> Logical Operator/2
  X/1 -> Half Adder/1(X)
  Half Adder 1/1(S) -> S/1
  Logical Operator/1 -> C/1

== system lab7_1/Subsystem3/Full Adder1 ==
  X : Inport
  Y : Inport  Port=2
  Z : Inport  Port=3
  Half Adder : Subsystem
  Half Adder 1 : Subsystem
  Logical Operator : Logic  Operator=OR  IconShape=distinctive  AllPortsSameDT=off  OutDataTypeStr=boolean
  S : Outport
  C : Outport  Port=2
  wires:
  Half Adder/1(S) -> Half Adder 1/1(X)
  Y/1 -> Half Adder/2(Y)
  Half Adder 1/2(C) -> Logical Operator/1
  Z/1 -> Half Adder 1/2(Y)
  Half Adder/2(C) -> Logical Operator/2
  X/1 -> Half Adder/1(X)
  Half Adder 1/1(S) -> S/1
  Logical Operator/1 -> C/1

== system lab7_1/Subsystem3/Full Adder2 ==
  X : Inport
  Y : Inport  Port=2
  Z : Inport  Port=3
  Half Adder : Subsystem
  Half Adder 1 : Subsystem
  Logical Operator : Logic  Operator=OR  IconShape=distinctive  AllPortsSameDT=off  OutDataTypeStr=boolean
  S : Outport
  C : Outport  Port=2
  wires:
  Half Adder/1(S) -> Half Adder 1/1(X)
  Y/1 -> Half Adder/2(Y)
  Half Adder 1/2(C) -> Logical Operator/1
  Z/1 -> Half Adder 1/2(Y)
  Half Adder/2(C) -> Logical Operator/2
  X/1 -> Half Adder/1(X)
  Half Adder 1/1(S) -> S/1
  Logical Operator/1 -> C/1

== system lab7_1/Subsystem3/Full Adder3 ==
  X : Inport
  Y : Inport  Port=2
  Z : Inport  Port=3
  Half Adder : Subsystem
  Half Adder 1 : Subsystem
  Logical Operator : Logic  Operator=OR  IconShape=distinctive  AllPortsSameDT=off  OutDataTypeStr=boolean
  S : Outport
  C : Outport  Port=2
  wires:
  Half Adder/1(S) -> Half Adder 1/1(X)
  Y/1 -> Half Adder/2(Y)
  Half Adder 1/2(C) -> Logical Operator/1
  Z/1 -> Half Adder 1/2(Y)
  Half Adder/2(C) -> Logical Operator/2
  X/1 -> Half Adder/1(X)
  Half Adder 1/1(S) -> S/1
  Logical Operator/1 -> C/1

== system lab7_1/Subsystem3/Full Adder4 ==
  X : Inport
  Y : Inport  Port=2
  Z : Inport  Port=3
  Half Adder : Subsystem
  Half Adder 1 : Subsystem
  Logical Operator : Logic  Operator=OR  IconShape=distinctive  AllPortsSameDT=off  OutDataTypeStr=boolean
  S : Outport
  C : Outport  Port=2
  wires:
  Half Adder/1(S) -> Half Adder 1/1(X)
  Y/1 -> Half Adder/2(Y)
  Half Adder 1/2(C) -> Logical Operator/1
  Z/1 -> Half Adder 1/2(Y)
  Half Adder/2(C) -> Logical Operator/2
  X/1 -> Half Adder/1(X)
  Half Adder 1/1(S) -> S/1
  Logical Operator/1 -> C/1

== system lab7_1/Subsystem3/Full Adder5 ==
  X : Inport
  Y : Inport  Port=2
  Z : Inport  Port=3
  Half Adder : Subsystem
  Half Adder 1 : Subsystem
  Logical Operator : Logic  Operator=OR  IconShape=distinctive  AllPortsSameDT=off  OutDataTypeStr=boolean
  S : Outport
  C : Outport  Port=2
  wires:
  Half Adder/1(S) -> Half Adder 1/1(X)
  Y/1 -> Half Adder/2(Y)
  Half Adder 1/2(C) -> Logical Operator/1
  Z/1 -> Half Adder 1/2(Y)
  Half Adder/2(C) -> Logical Operator/2
  X/1 -> Half Adder/1(X)
  Half Adder 1/1(S) -> S/1
  Logical Operator/1 -> C/1

== system lab7_1/Subsystem3/Full Adder6 ==
  X : Inport
  Y : Inport  Port=2
  Z : Inport  Port=3
  Half Adder : Subsystem
  Half Adder 1 : Subsystem
  Logical Operator : Logic  Operator=OR  IconShape=distinctive  AllPortsSameDT=off  OutDataTypeStr=boolean
  S : Outport
  C : Outport  Port=2
  wires:
  Half Adder/1(S) -> Half Adder 1/1(X)
  Y/1 -> Half Adder/2(Y)
  Half Adder 1/2(C) -> Logical Operator/1
  Z/1 -> Half Adder 1/2(Y)
  Half Adder/2(C) -> Logical Operator/2
  X/1 -> Half Adder/1(X)
  Half Adder 1/1(S) -> S/1
  Logical Operator/1 -> C/1

== system lab7_1/Subsystem3/Full Adder7 ==
  X : Inport
  Y : Inport  Port=2
  Z : Inport  Port=3
  Half Adder : Subsystem
  Half Adder 1 : Subsystem
  Logical Operator : Logic  Operator=OR  IconShape=distinctive  AllPortsSameDT=off  OutDataTypeStr=boolean
  S : Outport
  C : Outport  Port=2
  wires:
  Half Adder/1(S) -> Half Adder 1/1(X)
  Y/1 -> Half Adder/2(Y)
  Half Adder 1/2(C) -> Logical Operator/1
  Z/1 -> Half Adder 1/2(Y)
  Half Adder/2(C) -> Logical Operator/2
  X/1 -> Half Adder/1(X)
  Half Adder 1/1(S) -> S/1
  Logical Operator/1 -> C/1

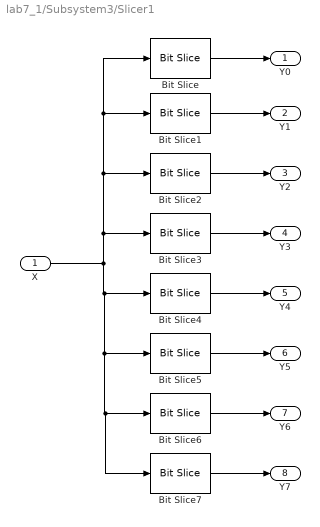
== system lab7_1/Subsystem3/Slicer1 ==
  X : Inport  OutDataTypeStr=int8  SampleTime=1
  Bit Slice : hdlsllib/Logic and Bit Operations/Bit Slice  lidx=7  ridx=7
  Bit Slice1 : hdlsllib/Logic and Bit Operations/Bit Slice  lidx=6  ridx=6
  Bit Slice2 : hdlsllib/Logic and Bit Operations/Bit Slice  lidx=5  ridx=5
  Bit Slice3 : hdlsllib/Logic and Bit Operations/Bit Slice  lidx=4  ridx=4
  Bit Slice4 : hdlsllib/Logic and Bit Operations/Bit Slice  lidx=3  ridx=3
  Bit Slice5 : hdlsllib/Logic and Bit Operations/Bit Slice  lidx=2  ridx=2
  Bit Slice6 : hdlsllib/Logic and Bit Operations/Bit Slice  lidx=1  ridx=1
  Bit Slice7 : hdlsllib/Logic and Bit Operations/Bit Slice  lidx=0  ridx=0
  Y0 : Outport
  Y1 : Outport  Port=2
  Y2 : Outport  Port=3
  Y3 : Outport  Port=4
  Y4 : Outport  Port=5
  Y5 : Outport  Port=6
  Y6 : Outport  Port=7
  Y7 : Outport  Port=8
  wires:
  Bit Slice1/1 -> Y1/1
  Bit Slice7/1 -> Y7/1
  X/1 -> Bit Slice7/1, Bit Slice6/1, Bit Slice5/1, Bit Slice4/1, Bit Slice3/1, Bit Slice2/1, Bit Slice1/1, Bit Slice/1
  Bit Slice/1 -> Y0/1
  Bit Slice4/1 -> Y4/1
  Bit Slice2/1 -> Y2/1
  Bit Slice5/1 -> Y5/1
  Bit Slice3/1 -> Y3/1
  Bit Slice6/1 -> Y6/1

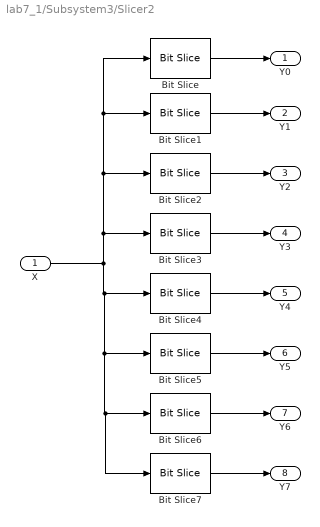
== system lab7_1/Subsystem3/Slicer2 ==
  X : Inport  OutDataTypeStr=int8  SampleTime=1
  Bit Slice : hdlsllib/Logic and Bit Operations/Bit Slice  lidx=7  ridx=7
  Bit Slice1 : hdlsllib/Logic and Bit Operations/Bit Slice  lidx=6  ridx=6
  Bit Slice2 : hdlsllib/Logic and Bit Operations/Bit Slice  lidx=5  ridx=5
  Bit Slice3 : hdlsllib/Logic and Bit Operations/Bit Slice  lidx=4  ridx=4
  Bit Slice4 : hdlsllib/Logic and Bit Operations/Bit Slice  lidx=3  ridx=3
  Bit Slice5 : hdlsllib/Logic and Bit Operations/Bit Slice  lidx=2  ridx=2
  Bit Slice6 : hdlsllib/Logic and Bit Operations/Bit Slice  lidx=1  ridx=1
  Bit Slice7 : hdlsllib/Logic and Bit Operations/Bit Slice  lidx=0  ridx=0
  Y0 : Outport
  Y1 : Outport  Port=2
  Y2 : Outport  Port=3
  Y3 : Outport  Port=4
  Y4 : Outport  Port=5
  Y5 : Outport  Port=6
  Y6 : Outport  Port=7
  Y7 : Outport  Port=8
  wires:
  Bit Slice1/1 -> Y1/1
  Bit Slice7/1 -> Y7/1
  X/1 -> Bit Slice7/1, Bit Slice6/1, Bit Slice5/1, Bit Slice4/1, Bit Slice3/1, Bit Slice2/1, Bit Slice1/1, Bit Slice/1
  Bit Slice/1 -> Y0/1
  Bit Slice4/1 -> Y4/1
  Bit Slice2/1 -> Y2/1
  Bit Slice5/1 -> Y5/1
  Bit Slice3/1 -> Y3/1
  Bit Slice6/1 -> Y6/1

== system lab7_1/Subsystem/Full Adder/Half Adder ==
  note: Subsystem
  X : Inport
  Y : Inport  Port=2
  Logical Operator : Logic  IconShape=distinctive  AllPortsSameDT=off  OutDataTypeStr=boolean
  Logical Operator1 : Logic  Operator=XOR  IconShape=distinctive  AllPortsSameDT=off  OutDataTypeStr=boolean
  S : Outport
  C : Outport  Port=2
  wires:
  X/1 -> Logical Operator/1, Logical Operator1/1
  Y/1 -> Logical Operator1/2, Logical Operator/2
  Logical Operator/1 -> C/1
  Logical Operator1/1 -> S/1

== system lab7_1/Subsystem/Full Adder/Half Adder 1 ==
  note: Subsystem
  X : Inport
  Y : Inport  Port=2
  Logical Operator : Logic  IconShape=distinctive  AllPortsSameDT=off  OutDataTypeStr=boolean
  Logical Operator1 : Logic  Operator=XOR  IconShape=distinctive  AllPortsSameDT=off  OutDataTypeStr=boolean
  S : Outport
  C : Outport  Port=2
  wires:
  X/1 -> Logical Operator/1, Logical Operator1/1
  Y/1 -> Logical Operator1/2, Logical Operator/2
  Logical Operator/1 -> C/1
  Logical Operator1/1 -> S/1

== system lab7_1/Subsystem/Full Adder1/Half Adder ==
  note: Subsystem
  X : Inport
  Y : Inport  Port=2
  Logical Operator : Logic  IconShape=distinctive  AllPortsSameDT=off  OutDataTypeStr=boolean
  Logical Operator1 : Logic  Operator=XOR  IconShape=distinctive  AllPortsSameDT=off  OutDataTypeStr=boolean
  S : Outport
  C : Outport  Port=2
  wires:
  X/1 -> Logical Operator/1, Logical Operator1/1
  Y/1 -> Logical Operator1/2, Logical Operator/2
  Logical Operator/1 -> C/1
  Logical Operator1/1 -> S/1

== system lab7_1/Subsystem/Full Adder1/Half Adder 1 ==
  note: Subsystem
  X : Inport
  Y : Inport  Port=2
  Logical Operator : Logic  IconShape=distinctive  AllPortsSameDT=off  OutDataTypeStr=boolean
  Logical Operator1 : Logic  Operator=XOR  IconShape=distinctive  AllPortsSameDT=off  OutDataTypeStr=boolean
  S : Outport
  C : Outport  Port=2
  wires:
  X/1 -> Logical Operator/1, Logical Operator1/1
  Y/1 -> Logical Operator1/2, Logical Operator/2
  Logical Operator/1 -> C/1
  Logical Operator1/1 -> S/1

== system lab7_1/Subsystem/Full Adder2/Half Adder ==
  note: Subsystem
  X : Inport
  Y : Inport  Port=2
  Logical Operator : Logic  IconShape=distinctive  AllPortsSameDT=off  OutDataTypeStr=boolean
  Logical Operator1 : Logic  Operator=XOR  IconShape=distinctive  AllPortsSameDT=off  OutDataTypeStr=boolean
  S : Outport
  C : Outport  Port=2
  wires:
  X/1 -> Logical Operator/1, Logical Operator1/1
  Y/1 -> Logical Operator1/2, Logical Operator/2
  Logical Operator/1 -> C/1
  Logical Operator1/1 -> S/1

== system lab7_1/Subsystem/Full Adder2/Half Adder 1 ==
  note: Subsystem
  X : Inport
  Y : Inport  Port=2
  Logical Operator : Logic  IconShape=distinctive  AllPortsSameDT=off  OutDataTypeStr=boolean
  Logical Operator1 : Logic  Operator=XOR  IconShape=distinctive  AllPortsSameDT=off  OutDataTypeStr=boolean
  S : Outport
  C : Outport  Port=2
  wires:
  X/1 -> Logical Operator/1, Logical Operator1/1
  Y/1 -> Logical Operator1/2, Logical Operator/2
  Logical Operator/1 -> C/1
  Logical Operator1/1 -> S/1

== system lab7_1/Subsystem/Full Adder3/Half Adder ==
  note: Subsystem
  X : Inport
  Y : Inport  Port=2
  Logical Operator : Logic  IconShape=distinctive  AllPortsSameDT=off  OutDataTypeStr=boolean
  Logical Operator1 : Logic  Operator=XOR  IconShape=distinctive  AllPortsSameDT=off  OutDataTypeStr=boolean
  S : Outport
  C : Outport  Port=2
  wires:
  X/1 -> Logical Operator/1, Logical Operator1/1
  Y/1 -> Logical Operator1/2, Logical Operator/2
  Logical Operator/1 -> C/1
  Logical Operator1/1 -> S/1

== system lab7_1/Subsystem/Full Adder3/Half Adder 1 ==
  note: Subsystem
  X : Inport
  Y : Inport  Port=2
  Logical Operator : Logic  IconShape=distinctive  AllPortsSameDT=off  OutDataTypeStr=boolean
  Logical Operator1 : Logic  Operator=XOR  IconShape=distinctive  AllPortsSameDT=off  OutDataTypeStr=boolean
  S : Outport
  C : Outport  Port=2
  wires:
  X/1 -> Logical Operator/1, Logical Operator1/1
  Y/1 -> Logical Operator1/2, Logical Operator/2
  Logical Operator/1 -> C/1
  Logical Operator1/1 -> S/1

== system lab7_1/Subsystem/Full Adder4/Half Adder ==
  note: Subsystem
  X : Inport
  Y : Inport  Port=2
  Logical Operator : Logic  IconShape=distinctive  AllPortsSameDT=off  OutDataTypeStr=boolean
  Logical Operator1 : Logic  Operator=XOR  IconShape=distinctive  AllPortsSameDT=off  OutDataTypeStr=boolean
  S : Outport
  C : Outport  Port=2
  wires:
  X/1 -> Logical Operator/1, Logical Operator1/1
  Y/1 -> Logical Operator1/2, Logical Operator/2
  Logical Operator/1 -> C/1
  Logical Operator1/1 -> S/1

== system lab7_1/Subsystem/Full Adder4/Half Adder 1 ==
  note: Subsystem
  X : Inport
  Y : Inport  Port=2
  Logical Operator : Logic  IconShape=distinctive  AllPortsSameDT=off  OutDataTypeStr=boolean
  Logical Operator1 : Logic  Operator=XOR  IconShape=distinctive  AllPortsSameDT=off  OutDataTypeStr=boolean
  S : Outport
  C : Outport  Port=2
  wires:
  X/1 -> Logical Operator/1, Logical Operator1/1
  Y/1 -> Logical Operator1/2, Logical Operator/2
  Logical Operator/1 -> C/1
  Logical Operator1/1 -> S/1

== system lab7_1/Subsystem/Full Adder5/Half Adder ==
  note: Subsystem
  X : Inport
  Y : Inport  Port=2
  Logical Operator : Logic  IconShape=distinctive  AllPortsSameDT=off  OutDataTypeStr=boolean
  Logical Operator1 : Logic  Operator=XOR  IconShape=distinctive  AllPortsSameDT=off  OutDataTypeStr=boolean
  S : Outport
  C : Outport  Port=2
  wires:
  X/1 -> Logical Operator/1, Logical Operator1/1
  Y/1 -> Logical Operator1/2, Logical Operator/2
  Logical Operator/1 -> C/1
  Logical Operator1/1 -> S/1

== system lab7_1/Subsystem/Full Adder5/Half Adder 1 ==
  note: Subsystem
  X : Inport
  Y : Inport  Port=2
  Logical Operator : Logic  IconShape=distinctive  AllPortsSameDT=off  OutDataTypeStr=boolean
  Logical Operator1 : Logic  Operator=XOR  IconShape=distinctive  AllPortsSameDT=off  OutDataTypeStr=boolean
  S : Outport
  C : Outport  Port=2
  wires:
  X/1 -> Logical Operator/1, Logical Operator1/1
  Y/1 -> Logical Operator1/2, Logical Operator/2
  Logical Operator/1 -> C/1
  Logical Operator1/1 -> S/1

== system lab7_1/Subsystem/Full Adder6/Half Adder ==
  note: Subsystem
  X : Inport
  Y : Inport  Port=2
  Logical Operator : Logic  IconShape=distinctive  AllPortsSameDT=off  OutDataTypeStr=boolean
  Logical Operator1 : Logic  Operator=XOR  IconShape=distinctive  AllPortsSameDT=off  OutDataTypeStr=boolean
  S : Outport
  C : Outport  Port=2
  wires:
  X/1 -> Logical Operator/1, Logical Operator1/1
  Y/1 -> Logical Operator1/2, Logical Operator/2
  Logical Operator/1 -> C/1
  Logical Operator1/1 -> S/1

== system lab7_1/Subsystem/Full Adder6/Half Adder 1 ==
  note: Subsystem
  X : Inport
  Y : Inport  Port=2
  Logical Operator : Logic  IconShape=distinctive  AllPortsSameDT=off  OutDataTypeStr=boolean
  Logical Operator1 : Logic  Operator=XOR  IconShape=distinctive  AllPortsSameDT=off  OutDataTypeStr=boolean
  S : Outport
  C : Outport  Port=2
  wires:
  X/1 -> Logical Operator/1, Logical Operator1/1
  Y/1 -> Logical Operator1/2, Logical Operator/2
  Logical Operator/1 -> C/1
  Logical Operator1/1 -> S/1

== system lab7_1/Subsystem/Full Adder7/Half Adder ==
  note: Subsystem
  X : Inport
  Y : Inport  Port=2
  Logical Operator : Logic  IconShape=distinctive  AllPortsSameDT=off  OutDataTypeStr=boolean
  Logical Operator1 : Logic  Operator=XOR  IconShape=distinctive  AllPortsSameDT=off  OutDataTypeStr=boolean
  S : Outport
  C : Outport  Port=2
  wires:
  X/1 -> Logical Operator/1, Logical Operator1/1
  Y/1 -> Logical Operator1/2, Logical Operator/2
  Logical Operator/1 -> C/1
  Logical Operator1/1 -> S/1

== system lab7_1/Subsystem/Full Adder7/Half Adder 1 ==
  note: Subsystem
  X : Inport
  Y : Inport  Port=2
  Logical Operator : Logic  IconShape=distinctive  AllPortsSameDT=off  OutDataTypeStr=boolean
  Logical Operator1 : Logic  Operator=XOR  IconShape=distinctive  AllPortsSameDT=off  OutDataTypeStr=boolean
  S : Outport
  C : Outport  Port=2
  wires:
  X/1 -> Logical Operator/1, Logical Operator1/1
  Y/1 -> Logical Operator1/2, Logical Operator/2
  Logical Operator/1 -> C/1
  Logical Operator1/1 -> S/1

== system lab7_1/Subsystem1/Full Adder/Half Adder ==
  note: Subsystem
  X : Inport
  Y : Inport  Port=2
  Logical Operator : Logic  IconShape=distinctive  AllPortsSameDT=off  OutDataTypeStr=boolean
  Logical Operator1 : Logic  Operator=XOR  IconShape=distinctive  AllPortsSameDT=off  OutDataTypeStr=boolean
  S : Outport
  C : Outport  Port=2
  wires:
  X/1 -> Logical Operator/1, Logical Operator1/1
  Y/1 -> Logical Operator1/2, Logical Operator/2
  Logical Operator/1 -> C/1
  Logical Operator1/1 -> S/1

== system lab7_1/Subsystem1/Full Adder/Half Adder 1 ==
  note: Subsystem
  X : Inport
  Y : Inport  Port=2
  Logical Operator : Logic  IconShape=distinctive  AllPortsSameDT=off  OutDataTypeStr=boolean
  Logical Operator1 : Logic  Operator=XOR  IconShape=distinctive  AllPortsSameDT=off  OutDataTypeStr=boolean
  S : Outport
  C : Outport  Port=2
  wires:
  X/1 -> Logical Operator/1, Logical Operator1/1
  Y/1 -> Logical Operator1/2, Logical Operator/2
  Logical Operator/1 -> C/1
  Logical Operator1/1 -> S/1

== system lab7_1/Subsystem1/Full Adder1/Half Adder ==
  note: Subsystem
  X : Inport
  Y : Inport  Port=2
  Logical Operator : Logic  IconShape=distinctive  AllPortsSameDT=off  OutDataTypeStr=boolean
  Logical Operator1 : Logic  Operator=XOR  IconShape=distinctive  AllPortsSameDT=off  OutDataTypeStr=boolean
  S : Outport
  C : Outport  Port=2
  wires:
  X/1 -> Logical Operator/1, Logical Operator1/1
  Y/1 -> Logical Operator1/2, Logical Operator/2
  Logical Operator/1 -> C/1
  Logical Operator1/1 -> S/1

== system lab7_1/Subsystem1/Full Adder1/Half Adder 1 ==
  note: Subsystem
  X : Inport
  Y : Inport  Port=2
  Logical Operator : Logic  IconShape=distinctive  AllPortsSameDT=off  OutDataTypeStr=boolean
  Logical Operator1 : Logic  Operator=XOR  IconShape=distinctive  AllPortsSameDT=off  OutDataTypeStr=boolean
  S : Outport
  C : Outport  Port=2
  wires:
  X/1 -> Logical Operator/1, Logical Operator1/1
  Y/1 -> Logical Operator1/2, Logical Operator/2
  Logical Operator/1 -> C/1
  Logical Operator1/1 -> S/1

== system lab7_1/Subsystem1/Full Adder2/Half Adder ==
  note: Subsystem
  X : Inport
  Y : Inport  Port=2
  Logical Operator : Logic  IconShape=distinctive  AllPortsSameDT=off  OutDataTypeStr=boolean
  Logical Operator1 : Logic  Operator=XOR  IconShape=distinctive  AllPortsSameDT=off  OutDataTypeStr=boolean
  S : Outport
  C : Outport  Port=2
  wires:
  X/1 -> Logical Operator/1, Logical Operator1/1
  Y/1 -> Logical Operator1/2, Logical Operator/2
  Logical Operator/1 -> C/1
  Logical Operator1/1 -> S/1
